simulink model "hw6Q2_model"  (R2021a)
settings: Solver=VariableStepAuto  StartTime=0.0  StopTime=time_end  RelTol=1e-3
values from neighbouring files (symbols this model uses):
  alpha = 60    [anthony_code.m]    (also in hw6Q2.m; hw6Q2_tony.m)
  G = 100    [anthony_code.m]    (also in hw6Q2.m; hw6Q2_tony.m)
  K_i = K_i_list(i)    [hw6Q1.m]    (also in hw6Q2.m = K_i_list(ii); hw6Q2_tony.m = K_i_list(kk); hw6Q3.m = 0.5)
  K_p = 1    [hw6Q1.m]    (also in hw6Q2.m = K_p_list(pp); hw6Q2_tony.m = K_p_list(kk); hw6Q3.m)
  m = 1000    [anthony_code.m]    (also in hw6Q2.m; hw6Q2_tony.m)
  z_0 = r_0 / (E / alpha * K_i) + K_p * r_0 / K_i    [hw6Q2.m]
settings Model: Creator=kaiyu  LastModifiedBy=kaiyu

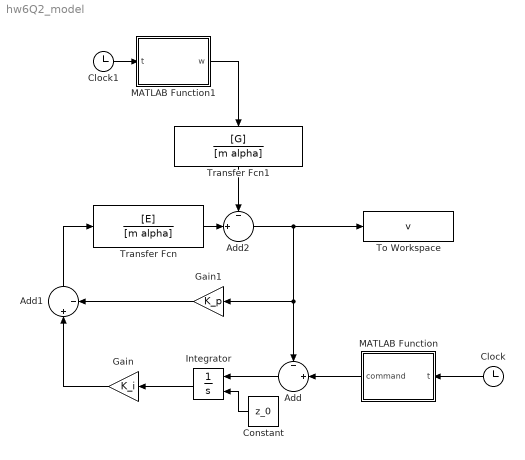
== system hw6Q2_model ==
  Add : Sum  Inputs=-|+||
  Add1 : Sum  Inputs=||+|-
  Add2 : Sum  Inputs=-|+||
  Clock : Clock
  Clock1 : Clock
  Constant : Constant  Value=z_0
  Gain : Gain  Gain=K_i
  Gain1 : Gain  Gain=K_p
  Integrator : Integrator  InitialConditionSource=external  InitialCondition=z_0
  MATLAB Function : MATLAB Function  TreatAsAtomicUnit=on
  MATLAB Function1 : MATLAB Function  TreatAsAtomicUnit=on
  To Workspace : ToWorkspace  VariableName=v  SaveFormat=Timeseries  SampleTime=-1
  Transfer Fcn : TransferFcn  Numerator=[E]  Denominator=[m alpha]
  Transfer Fcn1 : TransferFcn  Numerator=[G]  Denominator=[m alpha]
  wires:
  Clock/1 -> MATLAB Function/1(t)
  Transfer Fcn1/1 -> Add2/1
  Add1/1 -> Transfer Fcn/1
  MATLAB Function1/1(w) -> Transfer Fcn1/1
  MATLAB Function/1(command) -> Add/2
  Transfer Fcn/1 -> Add2/2
  Add2/1 -> Gain1/1, Add/1, To Workspace/1
  Add/1 -> Integrator/1
  Gain/1 -> Add1/1
  Integrator/1 -> Gain/1
  Gain1/1 -> Add1/2
  Clock1/1 -> MATLAB Function1/1(t)
  Constant/1 -> Integrator/2

== matlab function hw6Q2_model/MATLAB Function ==
  data: t input; command output
function command = v_des(t)
if (t >= 0) && (t < 5)
    r = 50;
elseif (t >= 5) && (t < 15)
    r = 55;
elseif (t >= 15) && (t < 25)
    r = 60;
elseif (t >= 25) && (t < 45)
    r = 60 - 4/3 * (t - 25);
else
    r = 45;
end
command = r;

== matlab function hw6Q2_model/MATLAB Function1 ==
  data: t input; w output
function w = disturbance(t)
if (t >= 0) && (t < 35)
    d = 0;
elseif (t >= 35) && (t < 45)
    d = 2.6;
elseif (t >= 45) && (t < 55)
    d = 0;
elseif (t >= 55) && (t < 70)
    d = 10;
else
    d = 0;
end

w = d;
